simulink model "cruise_control_practice"  (R2020a)
settings: Solver=VariableStepAuto  StartTime=0.0  StopTime=10  RelTol=1e-3
PostLoadFcn:
  | u=10;
  | m=0.05;
  | b=0.0015;
settings Model: Creator=Ganesh  LastModifiedBy=Ganesh

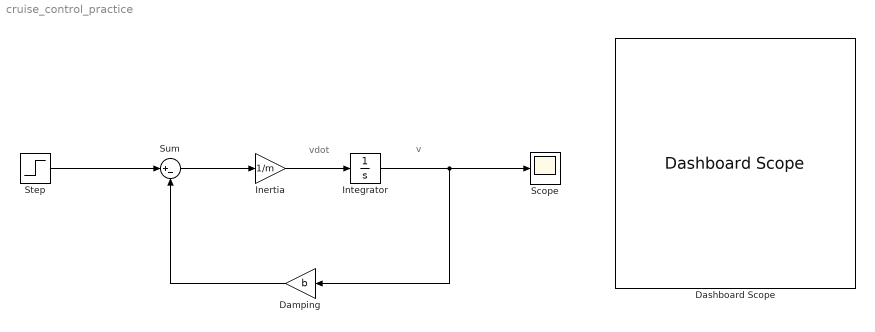
== system cruise_control_practice ==
  note: v
  note: vdot
  Damping : Gain  Gain=b
  Dashboard Scope : DashboardScope
  Inertia : Gain  Gain=1/m
  Integrator : Integrator
  Scope : Scope
  Step : Step  Time=5  After=u  SampleTime=0
  Sum : Sum  Inputs=|+-
  wires:
  Step/1 -> Sum/1
  Sum/1 -> Inertia/1
  Inertia/1 -> Integrator/1
  Damping/1 -> Sum/2
  Integrator/1 -> Scope/1, Damping/1
